simulink library "FirUp"  (R2022b)
settings: Solver=VariableStepAuto  StartTime=0.0  StopTime=10.0  RelTol=1e-3
undefined symbols (not defined in the file or in its folder): Row
libraries: HandyTextFile x9, FeaturePath x2, RTC x2, $bdroot x2, TuneVar x2, dspmlti4 x1, FirGeneric x1, TOP x1
settings Model: Creator=jb10849  LastModifiedBy=fz1054048
settings SolverCC: AlgebraicLoopSolver=TrustRegion
settings DebuggingCC: UnconnectedInputMsg=warning  UnconnectedOutputMsg=warning  UnconnectedLineMsg=warning  SFMachineParentedDataDiag=warning  ArithmeticOperatorsInVariantConditions=warning
settings ModelReferenceCC: EnableRefExpFcnMdlSchedulingChecks=on
settings SFSimCC: SimUseLocalCustomCode=off  CustomCodeUndefinedFunction=UseInterfaceOnly
settings RTWCC: RTWUseLocalCustomCode=off  DLArmComputeVersion=19.05
settings CodeAppCC: StateflowObjectComments=on

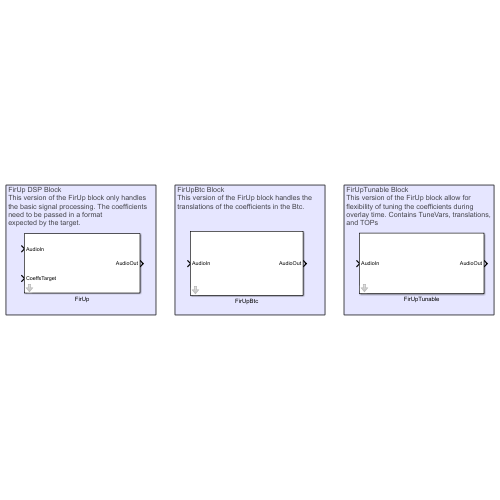
[thumbnail: Simulink's stored preview of the top-level diagram]
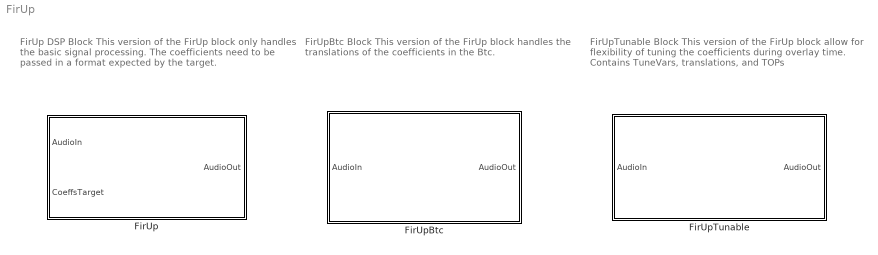
== system FirUp ==
  note: FirUp DSP Block
      | This version of the FirUp block only handles
      | the basic signal processing. The coefficients
      | need to be passed in a format
      | expected by the target.
  note: FirUpBtc Block
      | This version of the FirUp block handles the
      | translations of the coefficients in the Btc.
  note: FirUpTunable Block
      | This version of the FirUp block allow for
      | flexibility of tuning the coefficients during
      | overlay time. Contains TuneVars, translations,
      | and TOPs
  FirUp : Subsystem  mask(Blocklib FirUp){Config=[], FeatureName=FirUp}
      mask prompts: Config "FirUpConfig"; FeatureName "Feature path name:"
      mask init:
      | blkh=gcbh;
      | Config=BTConfig.Assert(blkh,Config);
      | 
      | Config.Validate();
      | Config.DoMaskInit(blkh);
      mask TypeOptions FeatureName: FeaturePath/FeatureName
      mask DialogControl ParamterGroupVar Prompt: Parameters
  FirUpBtc : Subsystem  mask(Blocklib FirUpBtc){Config=[], FeatureName=FirUpBtc}
      mask prompts: Config "FirUpBtcConfig"; FeatureName "Feature path name:"
      mask init:
      | blkh=gcbh;
      | Config=BTConfig.Assert(blkh,Config);
      | 
      | Config.Validate();
      | Config.DoMaskInit(blkh);
      mask TypeOptions FeatureName: FirUp/FeatureName
  FirUpTunable : Subsystem  mask(Blocklib FirUpTunable){Config=[], FeatureName=FirUpTunable}
      mask prompts: Config "FirUpTunableConfig"; FeatureName "Feature path name:"
      mask init:
      | blkh=gcbh;
      | Config=BTConfig.Assert(blkh,Config);
      | 
      | Config.Validate();
      | Config.DoMaskInit(blkh);
      mask TypeOptions FeatureName: FeaturePath/FeatureName

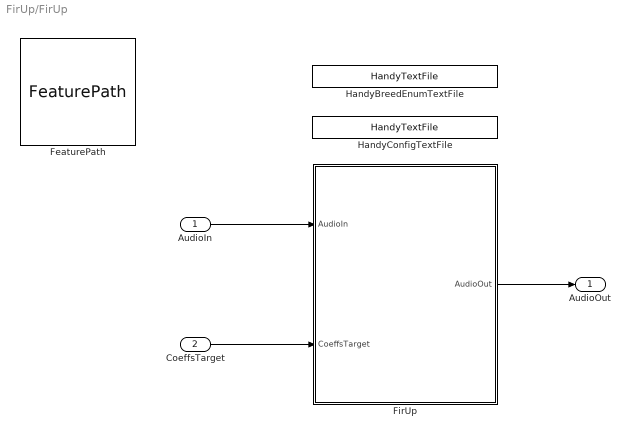
== system FirUp/FirUp ==
  AudioIn : Inport
  CoeffsTarget : Inport  Port=2
  FeaturePath : FeaturePath/FeaturePath  FeatureName=FirUp  IsGroup=off  GroupNumber=-1  IsModule=off  TriggerInit=[125 24 240 131]
      settings: SourceProductName=Bose Talaria
  FirUp : Subsystem  Variant=on
  HandyBreedEnumTextFile : HandyTextFile/HandyTextFile  TemplateSource=<dialog fields>  FileSuffix=BreedEnum  OpenDialogOnLoad=off  UseThisBlockName=off  AddGrandParentNamePrefix=off  TheDefaultText=% $(FILENAME) $(PREFIX) $(SUFFIX)  ShowInLibBrowser=on
      settings: SourceProductName=Bose Talaria
  HandyConfigTextFile : HandyTextFile/HandyTextFile  TemplateSource=Config  FileSuffix=File  OpenDialogOnLoad=off  UseThisBlockName=off  AddGrandParentNamePrefix=off  TheDefaultText=% $(FILENAME) $(PREFIX) $(SUFFIX)  ShowInLibBrowser=on
      settings: SourceProductName=Bose Talaria
  AudioOut : Outport
  wires:
  FirUp/1(AudioOut) -> AudioOut/1
  CoeffsTarget/1 -> FirUp/2(CoeffsTarget)
  AudioIn/1 -> FirUp/1(AudioIn)

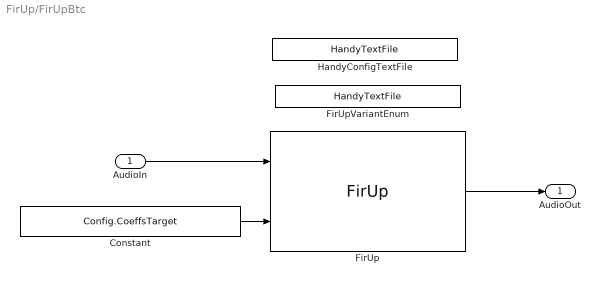
== system FirUp/FirUpBtc ==
  AudioIn : Inport
  Constant : Constant  Value=Config.CoeffsTarget  VectorParams1D=off  OutDataTypeStr=single
  FirUp : $bdroot/FirUp  Config=Config  FeatureName=FirUpBtc
  FirUpVariantEnum : HandyTextFile/HandyTextFile  TemplateSource=<dialog fields>  FileSuffix=VariantEnum  OpenDialogOnLoad=off  UseThisBlockName=on  AddGrandParentNamePrefix=off  TheDefaultText=% $(FILENAME) $(PREFIX) $(SUFFIX)  ShowInLibBrowser=on
      settings: SourceProductName=Bose Talaria
  HandyConfigTextFile : HandyTextFile/HandyTextFile  TemplateSource=Config  FileSuffix=File  OpenDialogOnLoad=off  UseThisBlockName=off  AddGrandParentNamePrefix=off  TheDefaultText=% $(FILENAME) $(PREFIX) $(SUFFIX)  ShowInLibBrowser=on
      settings: SourceProductName=Bose Talaria
  AudioOut : Outport
  wires:
  AudioIn/1 -> FirUp/1
  FirUp/1 -> AudioOut/1
  Constant/1 -> FirUp/2

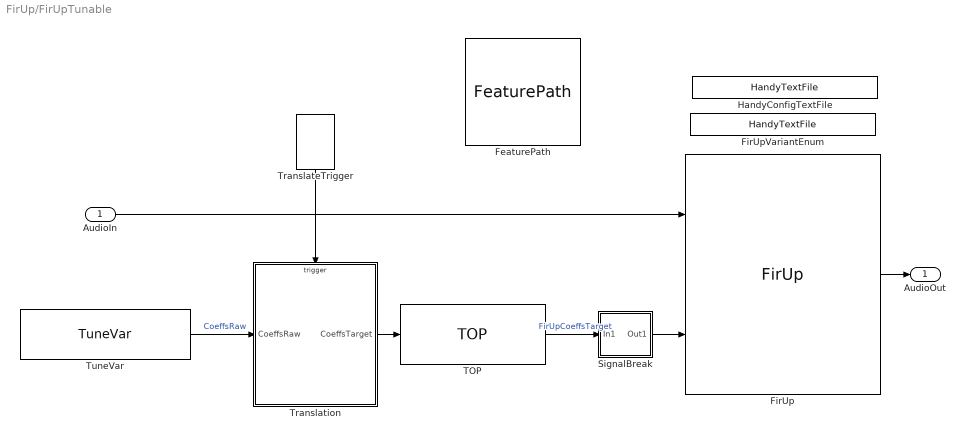
== system FirUp/FirUpTunable ==
  AudioIn : Inport
  FeaturePath : FeaturePath/FeaturePath  FeatureName=FirUpTunable  IsGroup=off  GroupNumber=-1  IsModule=off  TriggerInit=[15 -41 130 66]
      settings: SourceProductName=Bose Talaria
  FirUp : $bdroot/FirUp  Config=Config  FeatureName=FirUp
  FirUpVariantEnum : HandyTextFile/HandyTextFile  TemplateSource=<dialog fields>  FileSuffix=File  OpenDialogOnLoad=off  UseThisBlockName=off  AddGrandParentNamePrefix=off  TheDefaultText=% $(FILENAME) $(PREFIX) $(SUFFIX)  ShowInLibBrowser=on
      settings: SourceProductName=Bose Talaria
  HandyConfigTextFile : HandyTextFile/HandyTextFile  TemplateSource=Config  FileSuffix=File  OpenDialogOnLoad=off  UseThisBlockName=off  AddGrandParentNamePrefix=off  TheDefaultText=% $(FILENAME) $(PREFIX) $(SUFFIX)  ShowInLibBrowser=on
      settings: SourceProductName=Bose Talaria
  SignalBreak : Subsystem  Variant=on
  TOP : TOP/TOP  TriggerInit=[-50 225 95 285]  TopName=CoeffsTarget  DataTypeOut=Inherit: Same as input  BankNumber=0  PreOverlay=false  PostOverlay=Config.PostOverlayRequired  CompatibilityString=Config.Breed  Role=Automatic
      settings: SourceProductName=Bose Talaria
  TranslateTrigger : TuneVar/TranslateTrigger  TriggerInit=[-154 35 -116 90]
      settings: SourceProductName=Bose Talaria
  Translation : MATLAB Function  TreatAsAtomicUnit=on  mask(Talaria Translation){UpFactor=Config.UpFactor, Breed=Config.Breed}
      mask help: This MATLAB Function Block can be automatically inserted by several automation routines. Once placed, the block is ready to accept translation logic from the model designer.
  TuneVar : TuneVar/TuneVar  TuneName=CoeffsRaw  SpecifyMaxSize=off  VariableDim=1 (Row)  MaxSize=[1 1]  TunabilityNumber=1  MinValue=[]  MaxValue=[]  TriggerInit=[-430 230 -260 280]  MaskValue=Config.TuneVarCoeffsRaw
      settings: SourceProductName=Bose Talaria
  AudioOut : Outport
  wires:
  FirUp/1 -> AudioOut/1
  AudioIn/1 -> FirUp/1
  TranslateTrigger/1 -> Translation/Trigger
  TuneVar/1 -> Translation/1(CoeffsRaw)  "CoeffsRaw"
  Translation/1(CoeffsTarget) -> TOP/1
  TOP/1 -> SignalBreak/1(In1)  "FirUpCoeffsTarget"
  SignalBreak/1(Out1) -> FirUp/2

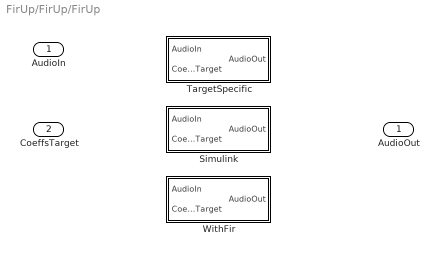
== system FirUp/FirUp/FirUp ==
  AudioIn : Inport
  CoeffsTarget : Inport  Port=2
  Simulink : Subsystem  VariantControl=(Config.Breed == AsdHwEnum.Simulink)
  TargetSpecific : Subsystem  VariantControl=((Config.Breed == AsdHwEnum.Generic) || (Config.Breed == AsdHwEnum.Hexagon)) && (Config.UseWithFirGeneric == false)
  WithFir : Subsystem  VariantControl=(default)
  AudioOut : Outport

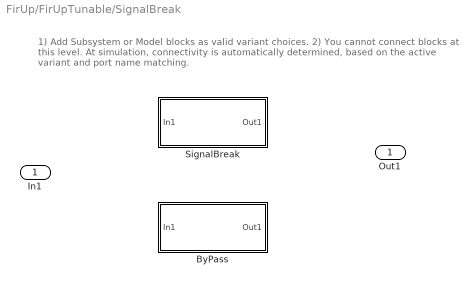
== system FirUp/FirUpTunable/SignalBreak ==
  note: 1) Add Subsystem or Model blocks as valid variant choices.
      | 2) You cannot connect blocks at this level. At simulation, connectivity is automatically
      | determined, based on the active variant and port name matching.
  In1 : Inport
  ByPass : Subsystem  VariantControl=(default)
  SignalBreak : Subsystem  VariantControl=(Config.Breed == AsdHwEnum.Hexagon)
  Out1 : Outport

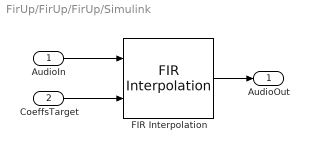
== system FirUp/FirUp/FirUp/Simulink ==
  AudioIn : Inport  OutDataTypeStr=single
  CoeffsTarget : Inport  Port=2  OutDataTypeStr=single
  FIR Interpolation : dspmlti4/FIR Interpolation  FilterSource=Input port  PrivateCoeffs=0  h=Config.Coefficients  L=Config.UpFactor  FilterObject=FINTERP  InputProcessing=Columns as channels (frame based)  framing=Enforce single-rate processing  outputBufInitCond=0  roundingMode=Floor  overflowMode=off  firstCoeffDataTypeStr=Inherit: Same word length as input  firstCoeffMin=[]  firstCoeffMax=[]  firstCoeffLastDataTypeStr=Inherit: Same word length as input  outputDataTypeStr=Inherit: Same as accumulator  outputMin=[]  outputMax=[]  outputLastDataTypeStr=Inherit: Same as accumulator
  AudioOut : Outport  OutDataTypeStr=single
  wires:
  AudioIn/1 -> FIR Interpolation/1
  FIR Interpolation/1 -> AudioOut/1
  CoeffsTarget/1 -> FIR Interpolation/2

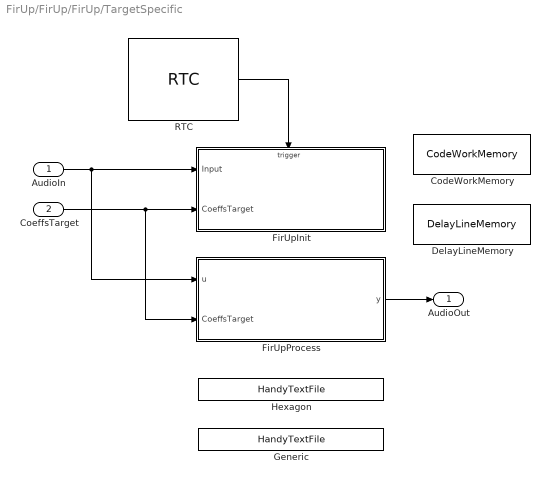
== system FirUp/FirUp/FirUp/TargetSpecific ==
  AudioIn : Inport
  CoeffsTarget : Inport  Port=2
  CodeWorkMemory : DataStoreMemory  DataStoreName=CodeWorkMemory  WriteAfterWriteMsg=warning  InitialValue=Config.BreedObj.CodeWorkMemoryInitValue  ShowAdditionalParam=off  OutDataTypeStr=uint32
  DelayLineMemory : DataStoreMemory  DataStoreName=DelayLineMemory  WriteAfterWriteMsg=warning  InitialValue=Config.BreedObj.DelayLineMemoryInitValue  ShowAdditionalParam=off  OutDataTypeStr=single
  FirUpInit : MATLAB Function  TreatAsAtomicUnit=on  mask{UpFactor=Config.UpFactor, Breed=Config.Breed}
  FirUpProcess : MATLAB Function  TreatAsAtomicUnit=on  mask{UpFactor=Config.UpFactor, Breed=Config.Breed}
  Generic : HandyTextFile/HandyTextFile  TemplateSource=<dialog fields>  FileSuffix=BreedConfig  OpenDialogOnLoad=off  UseThisBlockName=on  AddGrandParentNamePrefix=on  TheDefaultText=|  ShowInLibBrowser=on
      | % $(FILENAME) Setup model parameters for each "Init" callback (e.g. update diagram)
      | sample_rate_in_hertz = 44100;
      | frame_size = 32;
      | sysin_channel_count = 2;
      settings: SourceProductName=Bose Talaria
  Hexagon : HandyTextFile/HandyTextFile  TemplateSource=<dialog fields>  FileSuffix=BreedConfig  OpenDialogOnLoad=off  UseThisBlockName=on  AddGrandParentNamePrefix=on  TheDefaultText=|  ShowInLibBrowser=on
      | % $(FILENAME) Setup model parameters for each "Init" callback (e.g. update diagram)
      | sample_rate_in_hertz = 44100;
      | frame_size = 32;
      | sysin_channel_count = 2;
      settings: SourceProductName=Bose Talaria
  RTC : RTC/RTC  REQ_Priority=RTC_Mask.NormalPriority  RequestAtInit=on  EnableRequest=on  REQElemType1=uint32  REQElemWidth1=1  REQElemInitial1=[]  REQElemType2=uint32  REQElemWidth2=1  REQElemInitial2=[]  REQElemType3=uint32  REQElemWidth3=1  REQElemInitial3=[]  REQElemType4=uint32  REQElemWidth4=1  REQElemInitial4=[]  REQElemType5=uint32  REQElemWidth5=1  REQElemInitial5=[]  REQElemType6=uint32  REQElemWidth6=1  REQElemInitial6=[]  REQElemType7=uint32  REQElemWidth7=1  REQElemInitial7=[]  REQElemType8=uint32  REQElemWidth8=1  REQElemInitial8=[]  REQElemType9=uint32  REQElemWidth9=1  REQElemInitial9=[]  REQElemType10=uint32  REQElemWidth10=1  REQElemInitial10=[]  EnableResponse=off  EnableRSP_StatusIn=off  RSPElemType1=uint32  RSPElemWidth1=1  RSPElemType2=uint32  RSPElemWidth2=1  RSPElemType3=uint32  RSPElemWidth3=1  RSPElemType4=uint32  RSPElemWidth4=1  RSPElemType5=uint32  RSPElemWidth5=1  RSPElemType6=uint32  RSPElemWidth6=1  RSPElemType7=uint32  RSPElemWidth7=1  RSPElemType8=uint32  RSPElemWidth8=1  RSPElemType9=uint32  RSPElemWidth9=1  RSPElemType10=uint32  RSPElemWidth10=1  EnableNotification=off  EnableNTF_PrepTrig=off  NTFElemType1=uint32  NTFElemWidth1=1  NTFElemType2=uint32  NTFElemWidth2=1  NTFElemType3=uint32  NTFElemWidth3=1  NTFElemType4=uint32  NTFElemWidth4=1  NTFElemType5=uint32  NTFElemWidth5=1  NTFElemType6=uint32  NTFElemWidth6=1  NTFElemType7=uint32  NTFElemWidth7=1  NTFElemType8=uint32  NTFElemWidth8=1  NTFElemType9=uint32  NTFElemWidth9=1  NTFElemType10=uint32  NTFElemWidth10=1  MaskMessageName=InitReset
      settings: SourceProductName=Bose Talaria
  AudioOut : Outport
  wires:
  FirUpProcess/1(y) -> AudioOut/1
  RTC/1 -> FirUpInit/Trigger
  AudioIn/1 -> FirUpProcess/1(u), FirUpInit/1(Input)
  CoeffsTarget/1 -> FirUpProcess/2(CoeffsTarget), FirUpInit/2(CoeffsTarget)

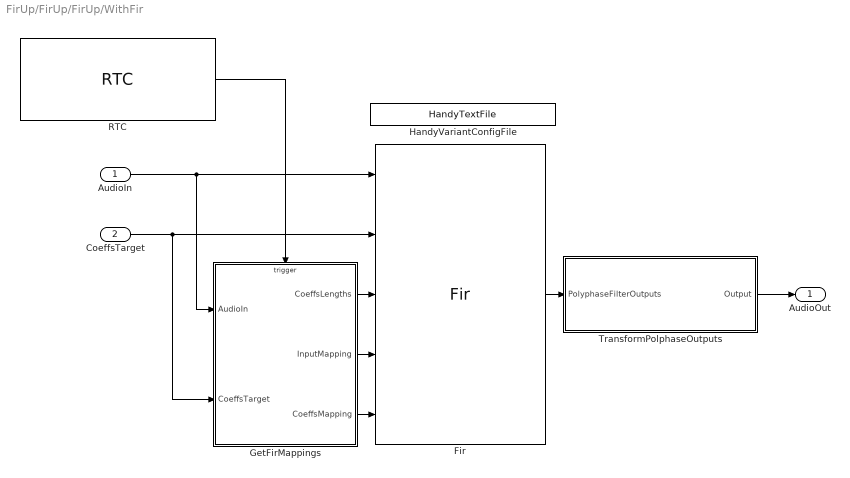
== system FirUp/FirUp/FirUp/WithFir ==
  AudioIn : Inport
  CoeffsTarget : Inport  Port=2
  Fir : FirGeneric/Fir  Config=Config.Fir  FeatureName=Fir
      settings: SourceProductName=Bose Blocklib
  GetFirMappings : MATLAB Function  TreatAsAtomicUnit=on  mask{UpFactor=Config.UpFactor}
  HandyVariantConfigFile : HandyTextFile/HandyTextFile  TemplateSource=<dialog fields>  FileSuffix=BreedConfig  OpenDialogOnLoad=off  UseThisBlockName=off  AddGrandParentNamePrefix=on  TheDefaultText=|  ShowInLibBrowser=on
      | % $(FILENAME) Setup model parameters for each "Init" callback (e.g. update diagram)
      | sample_rate_in_hertz = 44100;
      | frame_size = 32;
      | sysin_channel_count = 2;
      settings: SourceProductName=Bose Talaria
  RTC : RTC/RTC  REQ_Priority=RTC_Mask.NormalPriority  RequestAtInit=on  EnableRequest=on  REQElemType1=uint32  REQElemWidth1=1  REQElemInitial1=[]  REQElemType2=uint32  REQElemWidth2=1  REQElemInitial2=[]  REQElemType3=uint32  REQElemWidth3=1  REQElemInitial3=[]  REQElemType4=uint32  REQElemWidth4=1  REQElemInitial4=[]  REQElemType5=uint32  REQElemWidth5=1  REQElemInitial5=[]  REQElemType6=uint32  REQElemWidth6=1  REQElemInitial6=[]  REQElemType7=uint32  REQElemWidth7=1  REQElemInitial7=[]  REQElemType8=uint32  REQElemWidth8=1  REQElemInitial8=[]  REQElemType9=uint32  REQElemWidth9=1  REQElemInitial9=[]  REQElemType10=uint32  REQElemWidth10=1  REQElemInitial10=[]  EnableResponse=off  EnableRSP_StatusIn=off  RSPElemType1=uint32  RSPElemWidth1=1  RSPElemType2=uint32  RSPElemWidth2=1  RSPElemType3=uint32  RSPElemWidth3=1  RSPElemType4=uint32  RSPElemWidth4=1  RSPElemType5=uint32  RSPElemWidth5=1  RSPElemType6=uint32  RSPElemWidth6=1  RSPElemType7=uint32  RSPElemWidth7=1  RSPElemType8=uint32  RSPElemWidth8=1  RSPElemType9=uint32  RSPElemWidth9=1  RSPElemType10=uint32  RSPElemWidth10=1  EnableNotification=off  EnableNTF_PrepTrig=off  NTFElemType1=uint32  NTFElemWidth1=1  NTFElemType2=uint32  NTFElemWidth2=1  NTFElemType3=uint32  NTFElemWidth3=1  NTFElemType4=uint32  NTFElemWidth4=1  NTFElemType5=uint32  NTFElemWidth5=1  NTFElemType6=uint32  NTFElemWidth6=1  NTFElemType7=uint32  NTFElemWidth7=1  NTFElemType8=uint32  NTFElemWidth8=1  NTFElemType9=uint32  NTFElemWidth9=1  NTFElemType10=uint32  NTFElemWidth10=1  MaskMessageName=WithFirInitReset
      settings: SourceProductName=Bose Talaria
  TransformPolphaseOutputs : MATLAB Function  TreatAsAtomicUnit=on  mask{UpFactor=Config.UpFactor}
  AudioOut : Outport
  wires:
  GetFirMappings/1(CoeffsLengths) -> Fir/3
  GetFirMappings/3(CoeffsMapping) -> Fir/5
  GetFirMappings/2(InputMapping) -> Fir/4
  RTC/1 -> GetFirMappings/Trigger
  TransformPolphaseOutputs/1(Output) -> AudioOut/1
  CoeffsTarget/1 -> GetFirMappings/2(CoeffsTarget), Fir/2
  Fir/1 -> TransformPolphaseOutputs/1(PolyphaseFilterOutputs)
  AudioIn/1 -> GetFirMappings/1(AudioIn), Fir/1

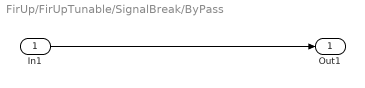
== system FirUp/FirUpTunable/SignalBreak/ByPass ==
  In1 : Inport
  Out1 : Outport
  wires:
  In1/1 -> Out1/1

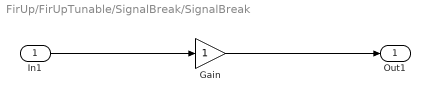
== system FirUp/FirUpTunable/SignalBreak/SignalBreak ==
  In1 : Inport
  Gain : Gain
  Out1 : Outport
  wires:
  In1/1 -> Gain/1
  Gain/1 -> Out1/1

== matlab function FirUp/FirUp/TargetSpecific/FirUpProcess ==
  data: u input; y output; UpFactor parameter; DelayLineMemory data_store_memory; CodeWorkMemory data_store_memory; Breed parameter; CoeffsTarget input
function y = FirUpProcess(u, UpFactor, Breed, CoeffsTarget)
% Upsample the input signal by an integer-valued factor, then apply an 
% FIR filter. 

global DelayLineMemory;
global CodeWorkMemory;

if(coder.target('MATLAB') || coder.target('Sfun')) 
    y = FirUpProcessSim(u, CoeffsTarget, UpFactor, true, Breed);
else
    switch(Breed)
        case(FirUpBreedEnum.Generic)
            y = firup_generic_process(single(u), single(DelayLineMemory), uint32(CodeWorkMemory), uint32(UpFactor));
        case(FirUpBreedEnum.Hexagon)
            y = firup_hexagon_process(single(u), single(DelayLineMemory), uint32(CodeWorkMemory), uint32(UpFactor));
    end
end
end

function y = firup_generic_process(u, DelayLineMemory, CodeWorkMemory, UpFactor)
coder.replace('-errorifnoreplacement');
[FrameSize, NumChannels] = size(u);
y = single(zeros(FrameSize*UpFactor, NumChannels));
end
function y = firup_hexagon_process(u, DelayLineMemory, CodeWorkMemory, UpFactor)
coder.replace('-errorifnoreplacement');
[FrameSize, NumChannels] = size(u);
y = single(zeros(FrameSize*UpFactor, NumChannels));
end

== matlab function FirUp/FirUp/TargetSpecific/FirUpInit ==
  data: Input input; UpFactor parameter; CodeWorkMemory data_store_memory; Breed parameter; CoeffsTarget input
  events: trigger input FUNCTION_CALL_EVENT
function FirUpInit(Input, UpFactor, Breed, CoeffsTarget)

global CodeWorkMemory;

[FrameSize, NumChannels] = size(Input);
FilterLength = numel(CoeffsTarget);
if(coder.target('MATLAB') || coder.target('Sfun')) 
    return;
else
    switch(Breed)
        case(FirUpBreedEnum.Generic)
            y = firup_generic_init(single(CoeffsTarget), uint32(FrameSize), uint32(UpFactor), uint32(FilterLength), uint32(NumChannels), uint32(CodeWorkMemory));
            % NOTE: The CRL mechanism requires an output for the function call,
            % and appears to be optimized out if that return value isn't used. 
            % This is a dummy operation to make sure CRL ends up in generated code
            CodeWorkMemory(1) = y;
        case(FirUpBreedEnum.Hexagon)
            y = firup_hexagon_init(single(CoeffsTarget), uint32(FrameSize), uint32(UpFactor), uint32(FilterLength), uint32(NumChannels), uint32(CodeWorkMemory));
            % NOTE: The CRL mechanism requires an output for the function call,
            % and appears to be optimized out if that return value isn't used. 
            % This is a dummy operation to make sure CRL ends up in generated code
            CodeWorkMemory(1) = y;
    end
end
end

function y = firup_generic_init(CoeffsTarget, FrameSize, UpFactor, FilterLength, NumChannels, CodeWorkMemory)
coder.replace('-warnifnoreplacement');
y = CodeWorkMemory(1) + 1;
end
function y = firup_hexagon_init(CoeffsTarget, FrameSize, UpFactor, FilterLength, NumChannels, CodeWorkMemory)
coder.replace('-errorifnoreplacement');
y = CodeWorkMemory(1) + 1;
end

== matlab function FirUp/FirUp/WithFir/GetFirMappings ==
  data: AudioIn input; CoeffsTarget input; CoeffsLengths output; InputMapping output; CoeffsMapping output; UpFactor parameter
  events: trigger input FUNCTION_CALL_EVENT
function [CoeffsLengths, InputMapping, CoeffsMapping] = GetFirMappings(AudioIn, CoeffsTarget, UpFactor)

[~, NumChannels] = size(AudioIn);
NumOutputs = UpFactor*NumChannels;

% Coefficients are equally divided up into [UpFactor] number of coefficient
% sets. 
CoeffsLengths = uint32(ceil(ones(1,UpFactor).*(numel(CoeffsTarget)/UpFactor)));
% CoeffsLengths = uint32(ceil(ones(1,NumOutputs).*(numel(CoeffsTarget)/UpFactor)));


% Output is mapped as follows, where UpFactor = L and NumChannels = Nc
% ix = 0: Nc - 1
%   iy = 0: L - 1
% fcn(Input[ix], Filter[iy]) = Output[ix*L + iy]
%
% CoeffsMapping = [0, 1, 2 ... L-1, 0, 1, 2 ... L-1 ...]
CoeffsMapping = uint32(mod(0:NumOutputs-1,UpFactor));
% InputMapping = [0 0 0 0 ... 1 1 1 1 ... 2 2 2 2 ... Nc-1 Nc-1 Nc-1 Nc-1 ...]
InputMapping = uint32(reshape(repmat(0:NumChannels-1,UpFactor,1),1,[])');

end

== matlab function FirUp/FirUp/WithFir/TransformPolphaseOutputs ==
  data: PolyphaseFilterOutputs input; Output output; UpFactor parameter
function Output = TransformPolyphaseOutputs(PolyphaseFilterOutputs, UpFactor)
% Converts polyphase filter outputs into standard filter outputs

% Instantiate output array
[FrameSizeIn, PolyphaseChannels] = size(PolyphaseFilterOutputs);
NumChannels = PolyphaseChannels/UpFactor;
Output = zeros(FrameSizeIn*UpFactor, PolyphaseChannels/UpFactor,'single');
for ch = 1: NumChannels
    % Commutation of polyphase subfilter outputs into a single upsampled
    % output
    Output(:,ch) = reshape(PolyphaseFilterOutputs(:,(ch-1)*UpFactor + (1:UpFactor))',1,[]);
end
end

== matlab function FirUp/FirUpTunable/Translation ==
  data: CoeffsTarget output; CoeffsRaw input; UpFactor parameter; Breed parameter
  events: trigger input FUNCTION_CALL_EVENT
function CoeffsTarget  = FirUpTranslationMfb(CoeffsRaw, UpFactor, Breed)
%#codegen

% ----- To access TuneVar maximum size, current size, and current value:
%   Note: TuneVar signals arrive with exposed variable size information.
%         The expressions below illustrate for the "Tune1" input argument.
%
%   size(Tune1.Value) : the maximum possible size of the Tune1 variable
%
%   Tune.Size   : the current size of *valid* data in Tune1.Value
%
%   Tune1.Size(1) : Number of rows present in Tune1 - this does not vary.
%
%   Tune1.Size(2) : Number of columns currently valid in Tune1 - this is
%       the variable part of size that can change (if allowed by TuneVar).
%
%   Tune1.Value : the current value of the tune variable... but end-padded 
%       to the maximum available size with undefined/invalid data.
%
%   numel(Tune1.Value) : another way of looking at the maximum number of
%       elements that could arrive in Tune1.Value
%
% ----- To register an error, use the following method (works like printf):
%   TranslateError( <format string>, <arguments ... )
%   ... this error will cause the build process to abort.
% ----- For warnings (works like printf):
%   TranslateWarning( <format string>, <arguments ... )
%   ... this warning will not set the translation engine error state.

% Set default value if arg not specified
CoeffsTarget = FirUpTranslation(CoeffsRaw.Value, UpFactor, Breed);

end
